simulink model "multiAgents2"  (Simulink 7.0)
settings: Solver=ode45  StartTime=0.0  StopTime=10  RelTol=1e-5
values from neighbouring files (symbols this model uses):
  k11 = 300    [example.m]    (also in initMultiAgents.m)
  k12 = 50    [example.m]    (also in initMultiAgents.m)
  k21 = 300    [example.m]    (also in initMultiAgents.m)
  k22 = 50    [example.m]    (also in initMultiAgents.m)
  zeta = [0 0 -100 -200 100 -200 -200 -400 0 -400 200 -400].'    [initMultiAgents.m]
settings Model: Creator=wizest  LastModifiedBy=wizest

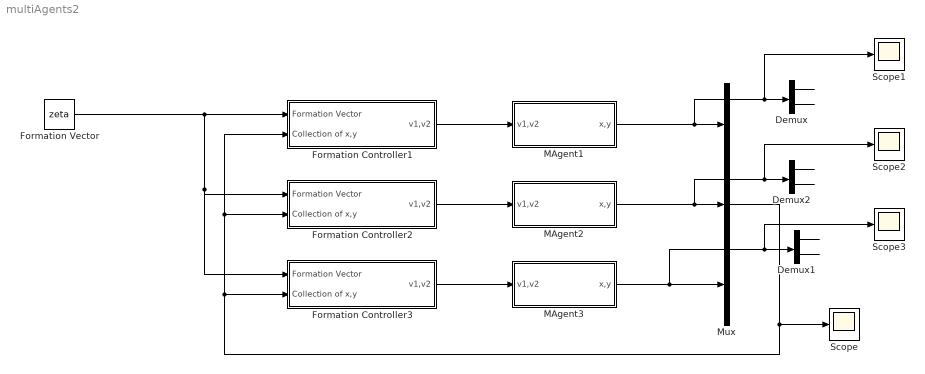
== system multiAgents2 ==
  Demux : Demux  Outputs=2
  Demux1 : Demux  Outputs=2
  Demux2 : Demux  Outputs=2
  Formation Controller1 : Subsystem
  Formation Controller2 : Subsystem
  Formation Controller3 : Subsystem
  Formation Vector : Constant  Value=zeta  OutDataType=sfix(16)  OutScaling=2^0
  MAgent1 : Subsystem
  MAgent2 : Subsystem
  MAgent3 : Subsystem
  Mux : Mux  Inputs=3
  Scope{,1..3} (4 alike) : Scope
      Scope settings: YMin=-1.75e+008  YMax=1.25e+008
      Scope1 settings: TimeRange=10  YMin=4  YMax=14
      Scope2 settings: TimeRange=10  YMin=-500000000000  YMax=3000000000000  SaveName=ScopeData3
      Scope3 settings: TimeRange=10  YMin=-3000000000000  YMax=500000000000  SaveName=ScopeData4
  wires:
  Formation Controller1/1(v1,v2) -> MAgent1/1(v1,v2)
  MAgent1/1(x,y) -> Mux/1, Demux/1, Scope1/1
  MAgent2/1(x,y) -> Mux/2, Demux2/1, Scope2/1
  MAgent3/1(x,y) -> Mux/3, Demux1/1, Scope3/1
  Formation Vector/1 -> Formation Controller1/1(Formation Vector), Formation Controller2/1(Formation Vector), Formation Controller3/1(Formation Vector)
  Formation Controller2/1(v1,v2) -> MAgent2/1(v1,v2)
  Formation Controller3/1(v1,v2) -> MAgent3/1(v1,v2)
  Mux/1 -> Scope/1, Formation Controller1/2(Collection of x,y), Formation Controller2/2(Collection of x,y), Formation Controller3/2(Collection of x,y)
  Demux/1 -> ?
  Demux/2 -> ?
  Demux1/1 -> ?
  Demux1/2 -> ?
  Demux2/1 -> ?
  Demux2/2 -> ?

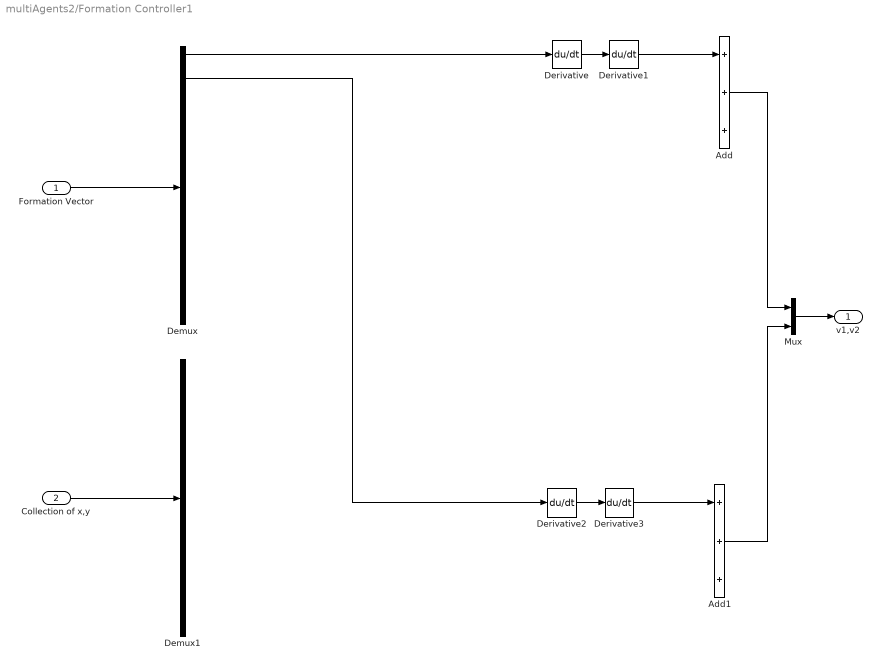
== system multiAgents2/Formation Controller1 ==
  Formation Vector : Inport  OutDataType=sfix(16)  OutScaling=2^0
  Collection of x,y : Inport  Port=2  OutDataType=sfix(16)  OutScaling=2^0
  Add : Sum  Inputs=+++  OutDataType=sfix(16)  OutScaling=2^-10
  Add1 : Sum  Inputs=+++  OutDataType=sfix(16)  OutScaling=2^-10
  Demux : Demux  Outputs=12
  Demux1 : Demux  Outputs=6
  Derivative{,1..3} (4 alike) : Derivative
  Mux : Mux  Inputs=2
  v1,v2 : Outport  OutDataType=sfix(16)  OutScaling=2^0
  wires:
  Formation Vector/1 -> Demux/1
  Collection of x,y/1 -> Demux1/1
  Derivative/1 -> Derivative1/1
  Derivative1/1 -> Add/1
  Demux/1 -> Derivative/1
  Derivative2/1 -> Derivative3/1
  Derivative3/1 -> Add1/1
  Demux/2 -> Derivative2/1
  Add1/1 -> Mux/2
  Add/1 -> Mux/1
  Mux/1 -> v1,v2/1

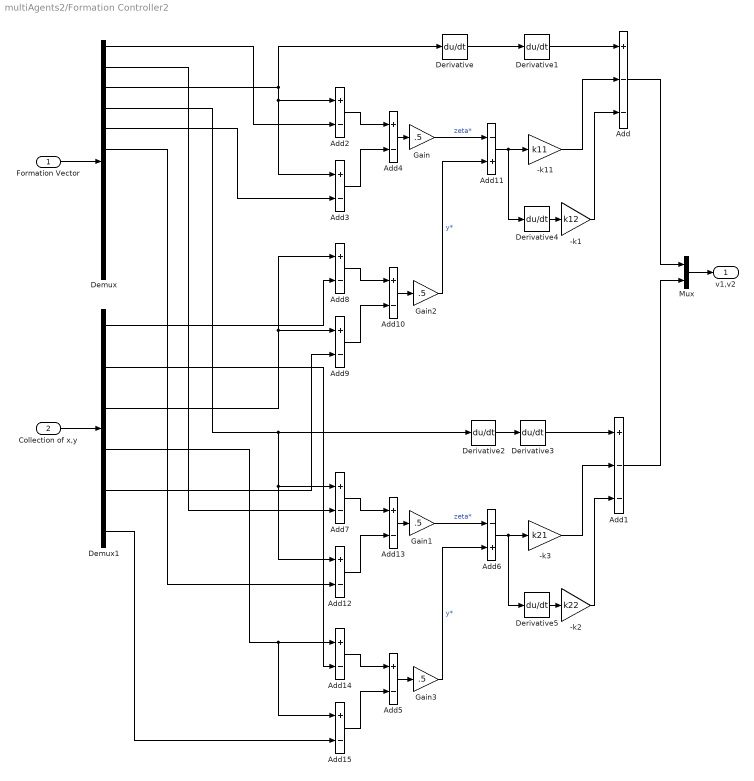
== system multiAgents2/Formation Controller2 ==
  Formation Vector : Inport  OutDataType=sfix(16)  OutScaling=2^0
  Collection of x,y : Inport  Port=2  OutDataType=sfix(16)  OutScaling=2^0
  -k1 : Gain  Gain=k12  ParameterDataType=sfix(16)  ParameterScaling=2^0  OutDataType=sfix(16)  OutScaling=2^0
  -k11 : Gain  Gain=k11  ParameterDataType=sfix(16)  ParameterScaling=2^0  OutDataType=sfix(16)  OutScaling=2^0
  -k2 : Gain  Gain=k22  ParameterDataType=sfix(16)  ParameterScaling=2^0  OutDataType=sfix(16)  OutScaling=2^0
  -k3 : Gain  Gain=k21  ParameterDataType=sfix(16)  ParameterScaling=2^0  OutDataType=sfix(16)  OutScaling=2^0
  Add : Sum  Inputs=+--  OutDataType=sfix(16)  OutScaling=2^-10
  Add1 : Sum  Inputs=+--  OutDataType=sfix(16)  OutScaling=2^-10
  Add{2..5,7..10,12..15} (12 alike) : Sum  Inputs=+-  OutDataType=sfix(16)  OutScaling=2^-10
  Add11 : Sum  Inputs=-+  OutDataType=sfix(16)  OutScaling=2^-10
  Add6 : Sum  Inputs=-+  OutDataType=sfix(16)  OutScaling=2^-10
  Demux : Demux  Outputs=12
  Demux1 : Demux  Outputs=6
  Derivative{,1..5} (6 alike) : Derivative
  Gain{,1..3} (4 alike) : Gain  Gain=.5  ParameterDataType=sfix(16)  ParameterScaling=2^0  OutDataType=sfix(16)  OutScaling=2^0
  Mux : Mux  Inputs=2
  v1,v2 : Outport  OutDataType=sfix(16)  OutScaling=2^0
  wires:
  Add1/1 -> Mux/2
  Derivative3/1 -> Add1/1
  Derivative2/1 -> Derivative3/1
  Add/1 -> Mux/1
  Mux/1 -> v1,v2/1
  Derivative1/1 -> Add/1
  Derivative/1 -> Derivative1/1
  Collection of x,y/1 -> Demux1/1
  Formation Vector/1 -> Demux/1
  Demux/4 -> Derivative2/1, Add7/1, Add12/1
  Demux/3 -> Derivative/1, Add2/1, Add3/1
  Add4/1 -> Gain/1
  Add2/1 -> Add4/1
  Add3/1 -> Add4/2
  -k11/1 -> Add/2
  -k1/1 -> Add/3
  Derivative4/1 -> -k1/1
  Demux/1 -> Add2/2
  Demux/5 -> Add3/2
  Add10/1 -> Gain2/1
  Add8/1 -> Add10/1
  Add9/1 -> Add10/2
  Demux1/3 -> Add8/1, Add9/1
  Demux1/1 -> Add8/2
  Demux1/5 -> Add9/2
  Gain2/1 -> Add11/2  "y*"
  Gain/1 -> Add11/1  "zeta*"
  Add11/1 -> -k11/1, Derivative4/1
  Add13/1 -> Gain1/1
  Add7/1 -> Add13/1
  Add12/1 -> Add13/2
  -k3/1 -> Add1/2
  -k2/1 -> Add1/3
  Derivative5/1 -> -k2/1
  Add5/1 -> Gain3/1
  Add14/1 -> Add5/1
  Add15/1 -> Add5/2
  Gain3/1 -> Add6/2  "y*"
  Gain1/1 -> Add6/1  "zeta*"
  Add6/1 -> Derivative5/1, -k3/1
  Demux1/4 -> Add14/1, Add15/1
  Demux/2 -> Add7/2
  Demux/6 -> Add12/2
  Demux1/2 -> Add14/2
  Demux1/6 -> Add15/2

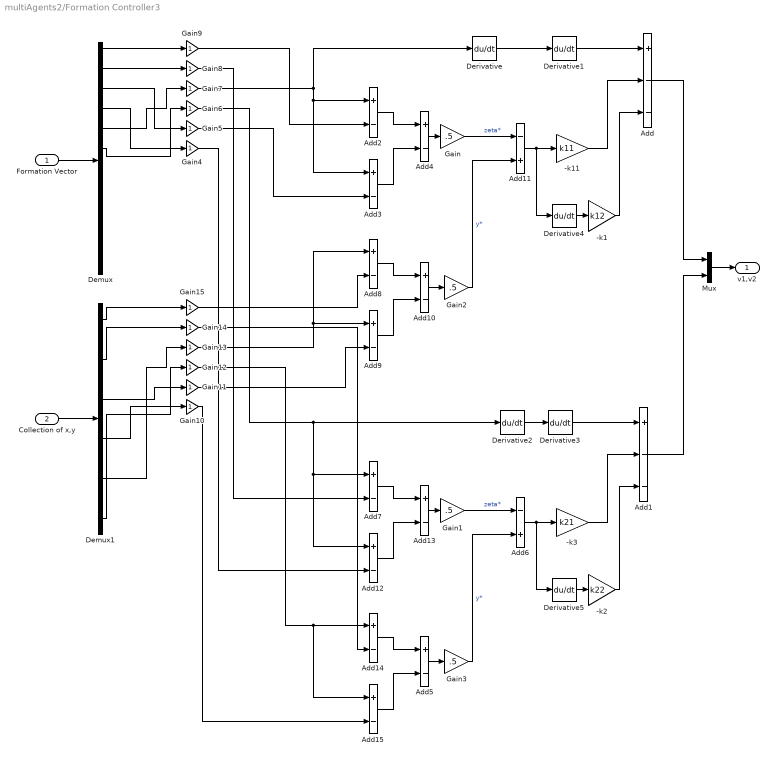
== system multiAgents2/Formation Controller3 ==
  Formation Vector : Inport  OutDataType=sfix(16)  OutScaling=2^0
  Collection of x,y : Inport  Port=2  OutDataType=sfix(16)  OutScaling=2^0
  -k1 : Gain  Gain=k12  ParameterDataType=sfix(16)  ParameterScaling=2^0  OutDataType=sfix(16)  OutScaling=2^0
  -k11 : Gain  Gain=k11  ParameterDataType=sfix(16)  ParameterScaling=2^0  OutDataType=sfix(16)  OutScaling=2^0
  -k2 : Gain  Gain=k22  ParameterDataType=sfix(16)  ParameterScaling=2^0  OutDataType=sfix(16)  OutScaling=2^0
  -k3 : Gain  Gain=k21  ParameterDataType=sfix(16)  ParameterScaling=2^0  OutDataType=sfix(16)  OutScaling=2^0
  Add : Sum  Inputs=+--  OutDataType=sfix(16)  OutScaling=2^-10
  Add1 : Sum  Inputs=+--  OutDataType=sfix(16)  OutScaling=2^-10
  Add{2..5,7..10,12..15} (12 alike) : Sum  Inputs=+-  OutDataType=sfix(16)  OutScaling=2^-10
  Add11 : Sum  Inputs=-+  OutDataType=sfix(16)  OutScaling=2^-10
  Add6 : Sum  Inputs=-+  OutDataType=sfix(16)  OutScaling=2^-10
  Demux : Demux  Outputs=12
  Demux1 : Demux  Outputs=6
  Derivative{,1..5} (6 alike) : Derivative
  Gain{,1..3} (4 alike) : Gain  Gain=.5  ParameterDataType=sfix(16)  ParameterScaling=2^0  OutDataType=sfix(16)  OutScaling=2^0
  Gain{4..15} (12 alike) : Gain  ParameterDataType=sfix(16)  ParameterScaling=2^0  OutDataType=sfix(16)  OutScaling=2^0
  Mux : Mux  Inputs=2
  v1,v2 : Outport  OutDataType=sfix(16)  OutScaling=2^0
  wires:
  Add6/1 -> -k3/1, Derivative5/1
  Gain1/1 -> Add6/1  "zeta*"
  Gain3/1 -> Add6/2  "y*"
  Add15/1 -> Add5/2
  Add14/1 -> Add5/1
  Add5/1 -> Gain3/1
  Derivative5/1 -> -k2/1
  -k2/1 -> Add1/3
  -k3/1 -> Add1/2
  Add12/1 -> Add13/2
  Add7/1 -> Add13/1
  Add13/1 -> Gain1/1
  Add11/1 -> Derivative4/1, -k11/1
  Gain/1 -> Add11/1  "zeta*"
  Gain2/1 -> Add11/2  "y*"
  Add9/1 -> Add10/2
  Add8/1 -> Add10/1
  Add10/1 -> Gain2/1
  Derivative4/1 -> -k1/1
  -k1/1 -> Add/3
  -k11/1 -> Add/2
  Add3/1 -> Add4/2
  Add2/1 -> Add4/1
  Add4/1 -> Gain/1
  Formation Vector/1 -> Demux/1
  Collection of x,y/1 -> Demux1/1
  Derivative/1 -> Derivative1/1
  Derivative1/1 -> Add/1
  Mux/1 -> v1,v2/1
  Add/1 -> Mux/1
  Derivative2/1 -> Derivative3/1
  Derivative3/1 -> Add1/1
  Add1/1 -> Mux/2
  Gain4/1 -> Add12/2
  Gain5/1 -> Add3/2
  Gain6/1 -> Add12/1, Add7/1, Derivative2/1
  Gain7/1 -> Add3/1, Add2/1, Derivative/1
  Gain8/1 -> Add7/2
  Gain9/1 -> Add2/2
  Gain10/1 -> Add15/2
  Gain11/1 -> Add9/2
  Gain12/1 -> Add15/1, Add14/1
  Gain13/1 -> Add9/1, Add8/1
  Gain14/1 -> Add14/2
  Gain15/1 -> Add8/2
  Demux/5 -> Gain7/1
  Demux/1 -> Gain9/1
  Demux/3 -> Gain5/1
  Demux/2 -> Gain8/1
  Demux/4 -> Gain4/1
  Demux/6 -> Gain6/1
  Demux1/5 -> Gain13/1
  Demux1/1 -> Gain15/1
  Demux1/3 -> Gain11/1
  Demux1/2 -> Gain14/1
  Demux1/4 -> Gain10/1
  Demux1/6 -> Gain12/1

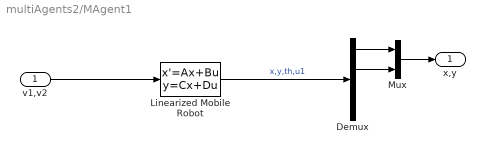
== system multiAgents2/MAgent1 ==
  v1,v2 : Inport  OutDataType=sfix(16)  OutScaling=2^0
  Demux : Demux
  Linearized Mobile Robot : StateSpace  A=[0 0 1 0; 0 0 0 1; 0 0 0 0; 0 0 0 0]  B=[0 0; 0 0; 1 0; 0 1]  C=eye(4)  D=[0 0;0 0 ;0 0;0 0]  X0=[5 5 (1)*cos(1) (1)*sin(1)]
  Mux : Mux  Inputs=2
  x,y : Outport  OutDataType=sfix(16)  OutScaling=2^0
  wires:
  Linearized Mobile Robot/1 -> Demux/1  "x,y,th,u1"
  v1,v2/1 -> Linearized Mobile Robot/1
  Demux/1 -> Mux/1
  Demux/2 -> Mux/2
  Mux/1 -> x,y/1

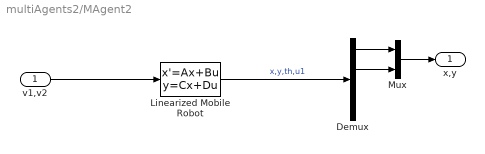
== system multiAgents2/MAgent2 ==
  v1,v2 : Inport  OutDataType=sfix(16)  OutScaling=2^0
  Demux : Demux
  Linearized Mobile Robot : StateSpace  A=[0 0 1 0; 0 0 0 1; 0 0 0 0; 0 0 0 0]  B=[0 0; 0 0; 1 0; 0 1]  C=eye(4)  D=[0 0;0 0 ;0 0;0 0]  X0=[-5 -5 (1)*cos(1) (1)*sin(1)]
  Mux : Mux  Inputs=2
  x,y : Outport  OutDataType=sfix(16)  OutScaling=2^0
  wires:
  Mux/1 -> x,y/1
  Demux/2 -> Mux/2
  Demux/1 -> Mux/1
  v1,v2/1 -> Linearized Mobile Robot/1
  Linearized Mobile Robot/1 -> Demux/1  "x,y,th,u1"

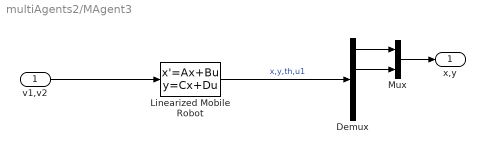
== system multiAgents2/MAgent3 ==
  v1,v2 : Inport  OutDataType=sfix(16)  OutScaling=2^0
  Demux : Demux
  Linearized Mobile Robot : StateSpace  A=[0 0 1 0; 0 0 0 1; 0 0 0 0; 0 0 0 0]  B=[0 0; 0 0; 1 0; 0 1]  C=eye(4)  D=[0 0;0 0 ;0 0;0 0]  X0=[0 0 (1)*cos(1) (1)*sin(1)]
  Mux : Mux  Inputs=2
  x,y : Outport  OutDataType=sfix(16)  OutScaling=2^0
  wires:
  Linearized Mobile Robot/1 -> Demux/1  "x,y,th,u1"
  v1,v2/1 -> Linearized Mobile Robot/1
  Demux/1 -> Mux/1
  Demux/2 -> Mux/2
  Mux/1 -> x,y/1
